simulink model "sim_notch440"  (R2020a)
settings: Solver=FixedStepDiscrete  StartTime=0.0  StopTime=0.75  FixedStep=6.25e-5  RelTol=1e-3
libraries: dspsrcs4 x1, dspvision x1
settings Model: Creator=ricar  LastModifiedBy=ricar

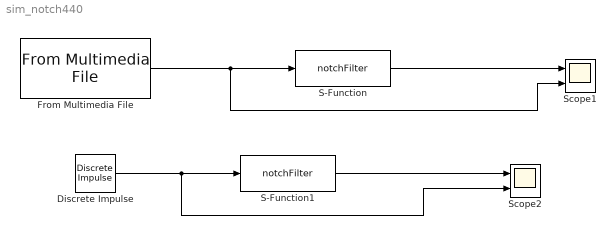
== system sim_notch440 ==
  Discrete Impulse : dspsrcs4/Discrete  Impulse  Delay=1000  SampleTime=1/16000  FrameSample=1  OutputFrames=off  dataType=double  isSigned=on  wordLen=16  udDataType=sfix(16)  fracBitsMode=Best precision  numFracBits=15  OutDataTypeStr=double  LastOutDataTypeStr=double
  From Multimedia File : dspvision/From Multimedia File  inputFilename=C:\Users\ricar\Desktop\Lab-DSP\lab3dsp_G6_Graves_Mardones\labC\sources\s-function_notch\alternate_tones_16_16.wav  readRange=[1 Inf]  loop=on  numPlays=inf  outputStreams=Audio only  videoDataType=single  audioDataType=double  inheritSampleTime=on  userDefinedSampleTime=1/30  noAudioOutput=off  isIntensityVideo=off  fourcc=RGB  colorVideoFormat=Separate color signals  outputEOF=off  dataOrg=Column-major  audioFrameSize=1  computeAudioFrameSize=off  outSamplingMode=Sample based
  S-Function : S-Function  FunctionName=notchFilter  SFunctionDeploymentMode=off  EnableBusSupport=off
  S-Function1 : S-Function  FunctionName=notchFilter  SFunctionDeploymentMode=off  EnableBusSupport=off
  Scope1 : Scope  NumInputPorts=2
  Scope2 : Scope  NumInputPorts=2
  wires:
  From Multimedia File/1 -> Scope1/2, S-Function/1
  S-Function/1 -> Scope1/1
  S-Function1/1 -> Scope2/1
  Discrete Impulse/1 -> Scope2/2, S-Function1/1
